simulink model "Frequency_Sampler"  (Simulink 9.2)
settings: Solver=ode23  StartTime=0.0  StopTime=100  RelTol=1e-3
undefined symbols (not defined in the file): ws, Xeo
settings Model: Creator=gyant  LastModifiedBy=gyant
settings DataIOCC: LimitDataPoints=off  SaveFormat=Dataset  SignalLoggingSaveFormat=Dataset
settings OptimizationCC: LifeSpan=auto
settings DebuggingCC: UnderspecifiedInitializationDetection=Simplified  MergeDetectMultiDrivingBlocksExec=error  FcnCallInpInsideContextMsg=error  StateNameClashWarn=none  SFUnexpectedBacktrackingDiag=error  SFNoUnconditionalDefaultTransitionDiag=error  SFExecutionAtInitializationDiag=warning
settings HardwareCC: ProdBitPerPointer=64  ProdBitPerSizeT=64  ProdBitPerPtrDiffT=64  ProdLargestAtomicFloat=Float  ProdIntDivRoundTo=Zero  ProdEndianess=LittleEndian  ProdWordSize=64  ProdHWDeviceType=Intel->x86-64 (Windows64)
settings ModelReferenceCC: PropagateSignalLabelsOutOfModel=on
settings SFSimCC: SimUseLocalCustomCode=on
settings RTWCC: RTWUseLocalCustomCode=on
settings CodeAppCC: StateflowObjectComments=off
settings GRTTargetCC: TargetLangStandard=C99 (ISO)  GeneratePreprocessorConditionals=Use local settings  CombineOutputUpdateFcns=on  GRTInterface=off
settings ConfigComp: CovMetricSettings=dwe  CovHtmlReporting=off  CovSaveCumulativeToWorkspaceVar=off  CovSaveSingleToWorkspaceVar=off  CovExternalEMLEnable=on

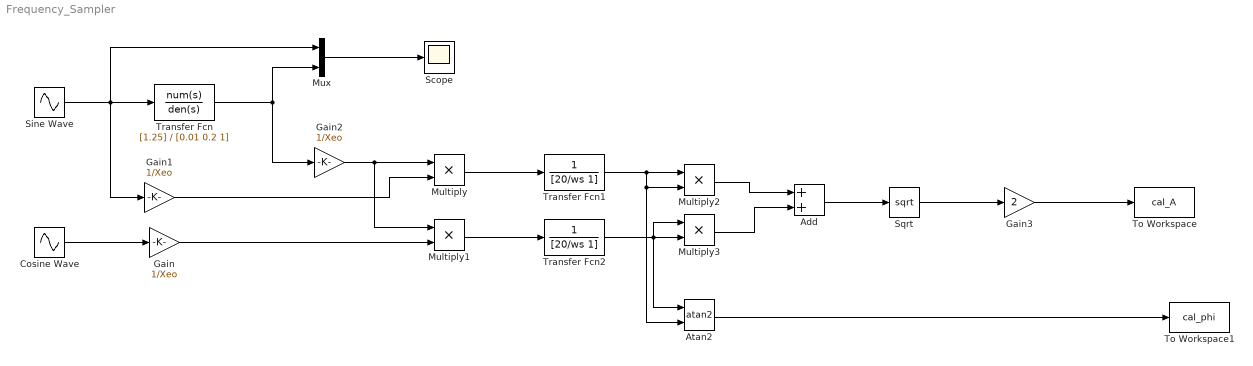
== system Frequency_Sampler ==
  Add : Sum
  Atan2 : Trigonometry  Operator=atan2
  Cosine Wave : Sin  Phase=pi/2  SampleTime=0
  Gain : Gain  Gain=1/Xeo
  Gain1 : Gain  Gain=1/Xeo
  Gain2 : Gain  Gain=1/Xeo
  Gain3 : Gain  Gain=2
  Multiply{,1..3} (4 alike) : Product
  Mux : Mux  Inputs=2
  Scope : Scope
  Sine Wave : Sin  SampleTime=0
  Sqrt : Sqrt  SaturateOnIntegerOverflow=on
  To Workspace : ToWorkspace  VariableName=cal_A  SaveFormat=Timeseries  SampleTime=-1
  To Workspace1 : ToWorkspace  VariableName=cal_phi  SaveFormat=Timeseries  SampleTime=-1
  Transfer Fcn : TransferFcn  Numerator=[1.25]  Denominator=[0.01 0.2 1]  ContinuousStateAttributes='Testsystem'
  Transfer Fcn1 : TransferFcn  Denominator=[20/ws 1]  ContinuousStateAttributes="''mean of r\""
  Transfer Fcn2 : TransferFcn  Denominator=[20/ws 1]
  wires:
  Cosine Wave/1 -> Gain/1
  Sine Wave/1 -> Gain1/1, Mux/1, Transfer Fcn/1
  Mux/1 -> Scope/1
  Transfer Fcn/1 -> Gain2/1, Mux/2
  Gain1/1 -> Multiply/2
  Gain2/1 -> Multiply/1, Multiply1/1
  Gain/1 -> Multiply1/2
  Multiply1/1 -> Transfer Fcn2/1
  Multiply/1 -> Transfer Fcn1/1
  Transfer Fcn1/1 -> Atan2/2, Multiply2/2, Multiply2/1
  Transfer Fcn2/1 -> Atan2/1, Multiply3/1, Multiply3/2
  Multiply2/1 -> Add/1
  Multiply3/1 -> Add/2
  Add/1 -> Sqrt/1
  Sqrt/1 -> Gain3/1
  Gain3/1 -> To Workspace/1
  Atan2/1 -> To Workspace1/1
